simulink model "Ideal_PV"  (R2026a)
settings: Solver=ode3  StopTime=0.6  FixedStep=0.01
libraries: simulink x1

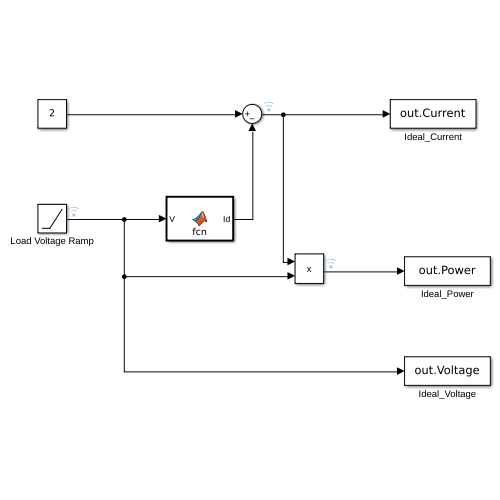
[thumbnail: Simulink's stored preview of the top-level diagram]
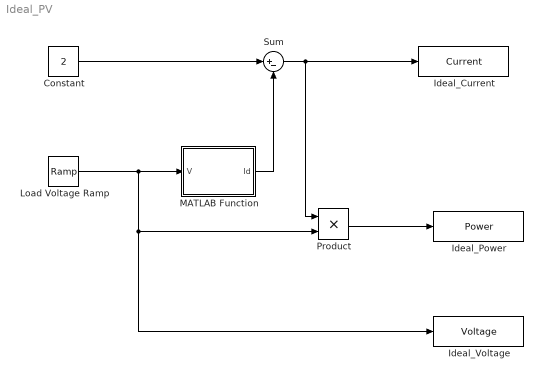
== system Ideal_PV ==
  Constant : Constant  Value=2
  Ideal_Current : ToWorkspace  VariableName=Current  SampleTime=-1
  Ideal_Power : ToWorkspace  VariableName=Power  SampleTime=-1
  Ideal_Voltage : ToWorkspace  VariableName=Voltage  SampleTime=-1
  Load Voltage Ramp : simulink/Sources/Ramp  slope=1  start=0  InitialOutput=0
  MATLAB Function : MATLAB Function  TreatAsAtomicUnit=on
  Product : Product
  Sum : Sum  Inputs=|+-
  wires:
  Constant/1 -> Sum/1
  MATLAB Function/1(Id) -> Sum/2
  Sum/1 -> Product/1, Ideal_Current/1
  Load Voltage Ramp/1 -> Ideal_Voltage/1, Product/2, MATLAB Function/1(V)
  Product/1 -> Ideal_Power/1

== matlab function Ideal_PV/MATLAB Function ==
  data: V input; Id output
function Id = fcn(V)
% Ideal diode current for single-diode PV model


I0 = 5.0e-10;     % reverse saturation current [A]
ad = 39.8;        % diode exponential constant [V^-1]

Id = I0*(exp(ad*V) - 1);
end
